simulink model "ECEF_2_ECI_test"  (R2016b)
settings: Solver=VariableStepAuto  StartTime=0.0  StopTime=1  RelTol=1e-3
values from neighbouring files (symbols this model uses):
  JD_tt_cent = 0.0426236319    [coord_rot_time_test_init.m]
  JD_ut1_cent = JD_2_cent*(JD2 - JD_J2000)    (= 0.0426236114155)    [coord_rot_time_test_init.m]
  rECEF = [ -1033.4793830; 7901.2952754; 6380.3565958 ]    [coord_rot_time_test_init.m]
  vECEF = [ -3.225636520; -2.872451450; 5.531924446 ]    [coord_rot_time_test_init.m]
libraries: coord_rotation_lib x1
settings Model: Creator=taylorreynolds  LastModifiedBy=taylorreynolds

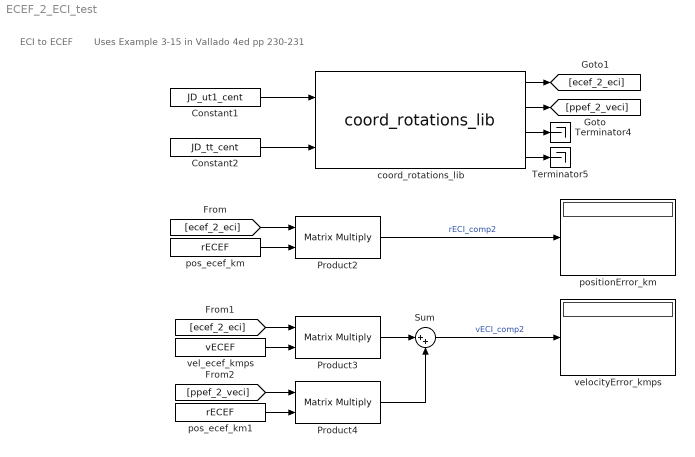
== system ECEF_2_ECI_test ==
  note: Uses Example 3-15 in Vallado 4ed pp 230-231
  note: ECI to ECEF
  Constant1 : Constant  Value=JD_ut1_cent
  Constant2 : Constant  Value=JD_tt_cent
  Product2 : Product  Multiplication=Matrix(*)
  Product3 : Product  Multiplication=Matrix(*)
  Product4 : Product  Multiplication=Matrix(*)
  Sum : Sum  Inputs=|++
  Terminator4 : Terminator
  Terminator5 : Terminator
  coord_rotations_lib : coord_rotation_lib/coord_rotations_lib
  pos_ecef_km : Constant  Value=rECEF
  pos_ecef_km1 : Constant  Value=rECEF
  positionError_km : Display
  vel_ecef_kmps : Constant  Value=vECEF
  velocityError_kmps : Display
  wires:
  Constant2/1 -> coord_rotations_lib/2
  Constant1/1 -> coord_rotations_lib/1
  pos_ecef_km/1 -> Product2/2
  vel_ecef_kmps/1 -> Product3/2
  Product2/1 -> positionError_km/1  "rECI_comp2"
  coord_rotations_lib/2 -> [ppef_2_veci]
  coord_rotations_lib/3 -> Terminator4/1
  coord_rotations_lib/4 -> Terminator5/1
  Sum/1 -> velocityError_kmps/1  "vECI_comp2"
  coord_rotations_lib/1 -> [ecef_2_eci]
  [ecef_2_eci] -> Product2/1
  [ecef_2_eci] -> Product3/1
  Product3/1 -> Sum/1
  pos_ecef_km1/1 -> Product4/2
  [ppef_2_veci] -> Product4/1
  Product4/1 -> Sum/2
